simulink model "mpcacc_second"  (Simulink 7.2)
settings: Solver=FixedStepDiscrete  StartTime=0.0  StopTime=36000  FixedStep=.1  RelTol=1e-3
InitFcn:
  | Ts = .1;
  | CruiseControl;
  | p1_params;
  | %Para_CYL52;
  | 
  | %self_ChangeDir;
  | Main_MPC_MTCACC1;
  | 
  | mpc_params;
  | LL_CtrlObj;
  | Ext_MPCpara;
  | Proc_RT_para;
undefined symbols (not defined in the file or in its folder): bit, Standard
libraries: xpclib x5
settings Model: Creator=ibm  LastModifiedBy=ddl  BufferReuse=off
settings OptimizationCC: BlockReduction=off  OptimizeBlockIOStorage=off  BufferReuse=off  ExpressionFolding=off  LocalBlockOutputs=off  InitFltsAndDblsToZero=on
settings DebuggingCC: SaveWithParameterizedLinksMsg=none
settings HardwareCC: ProdIntDivRoundTo=Zero  ProdEndianess=LittleEndian  ProdHWDeviceType=Generic->32-bit x86 compatible
settings RTWCC: SystemTargetFile=xpctarget.tlc  TemplateMakefile=xpc_vc.tmf  Description=xPC Target  ProcessScript=xpctarget_make_rtw_hook  RTWCompilerOptimization=On
settings xpcTargetCC: TargetFcnLib=ansi_tfl_table_tmw.mat  TargetFunctionLibrary=ANSI_C  PortableWordSizes=off  xPCisDownloadable=off

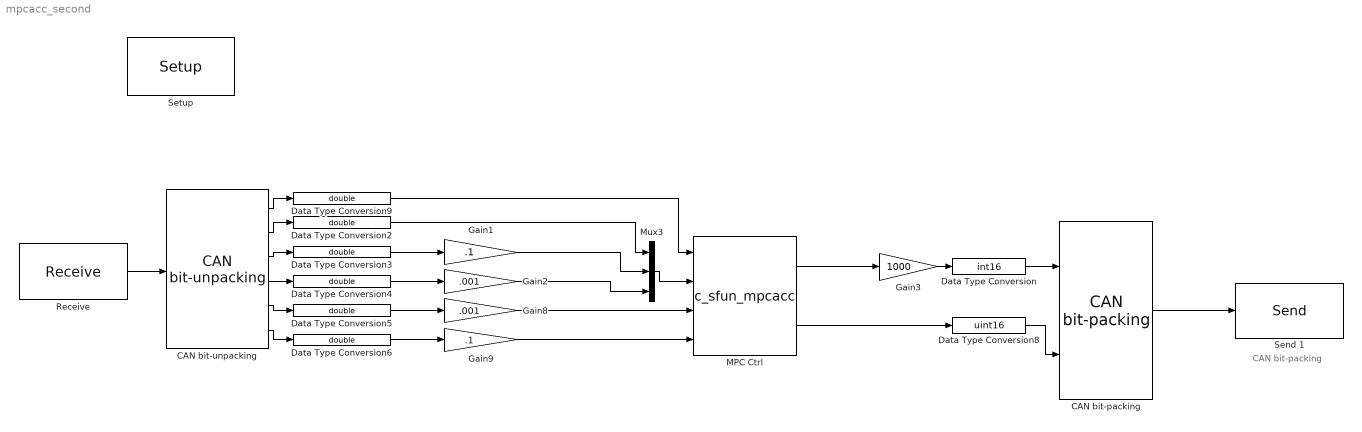
== system mpcacc_second ==
  note: CAN bit-packing
  "CAN bit-packing " : xpclib/CAN/Utilities/CAN bit-packing   bitpatterns={ [0:15],[16:31]}
  "CAN bit-unpacking " : xpclib/CAN/Utilities/CAN bit-unpacking   bitpatterns={ [0:7],[8:15],[16:23],[24,39],[40:55],[56:63] }  dtypes={ 'int8' ,'int8','int8','int16','int16','int8'}
  Data Type Conversion : DataTypeConversion  OutDataTypeMode=int16  OutDataType=sfix(16)  OutScaling=2^0  OutDataTypeStr=int16  RndMeth=Nearest  SaturateOnIntegerOverflow=on
  Data Type Conversion{2..6,9} (6 alike) : DataTypeConversion  OutDataTypeMode=double  OutDataType=sfix(16)  OutScaling=2^0  OutDataTypeStr=double
  Data Type Conversion8 : DataTypeConversion  OutDataTypeMode=uint16  OutDataType=sfix(16)  OutScaling=2^0  OutDataTypeStr=uint16  RndMeth=Nearest  SaturateOnIntegerOverflow=on
  Gain1 : Gain  Gain=.1  ParameterDataType=sfix(16)  ParameterScaling=2^0  OutDataType=sfix(16)  OutScaling=2^0
  Gain2 : Gain  Gain=.001  ParameterDataType=sfix(16)  ParameterScaling=2^0  OutDataType=sfix(16)  OutScaling=2^0
  Gain3 : Gain  Gain=1000  ParameterDataType=sfix(16)  ParameterScaling=2^0  OutDataType=sfix(16)  OutScaling=2^0
  Gain8 : Gain  Gain=.001  ParameterDataType=sfix(16)  ParameterScaling=2^0  OutDataType=sfix(16)  OutScaling=2^0
  Gain9 : Gain  Gain=.1  ParameterDataType=sfix(16)  ParameterScaling=2^0  OutDataType=sfix(16)  OutScaling=2^0
  MPC Ctrl : S-Function  FunctionName=c_sfun_mpcacc  Parameters="0.1, A, B, G, cofSVE, cofSDE, H,  Mctrl, T_u1, MT,  U_max, U_min, dU_max, dU_min, Y_max, Y_min,   D_safe, T_safe,  Xmin, aH, Hinv, TAB,  maxIter, A_cstrXmin  ,AHaH  ,AHS_uS_x  ,AHS_uSu1  ,AHS_uHv ,AHS_uSeH ,AHTduTu1 ,MYS_x ,MYSu1 ,MYHv ,MYSeH ,AsS_x ,AsSu1 ,AsHv ,AsSeH, AyS_x, AySu1, AyHv ,AySeH, AuTu1,S_uS_x, S_uSu1 ,S_uHv   ,S_uSeH ,TduTu1"  EnableBusSupport=off
  Mux3 : Mux  Inputs=3
  "Receive " : xpclib/CAN/Softing/CAN-AC2-104 SJA 1000/Receive   board=1  canPort=CAN 1  range=Standard (11-bit)  ids=[500]  output=Data  inten=on  ts=-1  ididx=[0]
  Send 1 : xpclib/CAN/Softing/CAN-AC2-104 SJA 1000/Send   board=1  canPort=CAN 1  range=Standard (11-bit)  ids=[501]  sizes=[8]  output=off  ts=-1  ididx=[0]
  "Setup " : xpclib/CAN/Softing/CAN-AC2-104 SJA 1000/Setup   board=1  can1Baudrate=500 kBaud  can1UserBR=[1,1,4,3]  can2Baudrate=500 kBaud  can2UserBR=[1,1,4,3]  init=[]  term=[]  ioBaseAddressL=0x240  memBaseAddressL=0xd0000  intNo=5
  wires:
  "Receive "/1 -> "CAN bit-unpacking "/1
  Data Type Conversion3/1 -> Gain1/1
  Data Type Conversion4/1 -> Gain2/1
  "CAN bit-packing "/1 -> Send 1/1
  Data Type Conversion/1 -> "CAN bit-packing "/1
  Data Type Conversion6/1 -> Gain9/1
  Data Type Conversion5/1 -> Gain8/1
  "CAN bit-unpacking "/1 -> Data Type Conversion9/1
  "CAN bit-unpacking "/2 -> Data Type Conversion2/1
  "CAN bit-unpacking "/3 -> Data Type Conversion3/1
  "CAN bit-unpacking "/4 -> Data Type Conversion4/1
  "CAN bit-unpacking "/5 -> Data Type Conversion5/1
  "CAN bit-unpacking "/6 -> Data Type Conversion6/1
  Mux3/1 -> MPC Ctrl/2
  Gain8/1 -> MPC Ctrl/3
  Gain9/1 -> MPC Ctrl/4
  Gain2/1 -> Mux3/3
  Gain1/1 -> Mux3/2
  Data Type Conversion2/1 -> Mux3/1
  Data Type Conversion9/1 -> MPC Ctrl/1
  MPC Ctrl/1 -> Gain3/1
  Data Type Conversion8/1 -> "CAN bit-packing "/2
  MPC Ctrl/2 -> Data Type Conversion8/1
  Gain3/1 -> Data Type Conversion/1
